simulink model "Fullmodelsimulation"  (R2017b)
settings: Solver=VariableStepAuto  StartTime=0.0  StopTime=inf  RelTol=1e-3
libraries: fullmodel x3
settings Model: Creator=minh  LastModifiedBy=minh

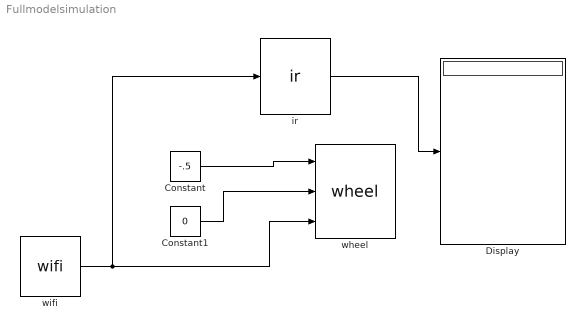
== system Fullmodelsimulation ==
  Constant : Constant  Value=-.5
  Constant1 : Constant  Value=0
  Display : Display
  "ir " : fullmodel/ir 
  wheel : fullmodel/wheel
  wifi : fullmodel/wifi
  wires:
  "ir "/1 -> Display/1
  wifi/1 -> wheel/3, "ir "/1
  Constant1/1 -> wheel/2
  Constant/1 -> wheel/1
